simulink model "Ground_Path"  (R2018a)
settings: Solver=ode1  StartTime=0.0  StopTime=constants.t_end  FixedStep=constants.dt  RelTol=1e-3  EnableMultiTasking=on
settings Model: ExtModeTrigDuration=5000  Creator=bruders  LastModifiedBy=Joseph
settings SolverCC: PositivePriorityOrder=on
settings DataIOCC: LimitDataPoints=on  SaveFormat=Array
settings OptimizationCC: LifeSpan=inf
settings DebuggingCC: SolverPrmCheckMsg=warning  AllowSymbolicDim=off  SFUnexpectedBacktrackingDiag=warning  SFNoUnconditionalDefaultTransitionDiag=warning  SFExecutionAtInitializationDiag=none
settings HardwareCC: ProdBitPerPointer=32  ProdBitPerSizeT=32  ProdBitPerPtrDiffT=32  ProdLargestAtomicFloat=None  ProdIntDivRoundTo=Undefined  ProdEndianess=Unspecified  ProdWordSize=32  ProdHWDeviceType=32-bit Generic
settings ModelReferenceCC: PropagateSignalLabelsOutOfModel=off
settings RTWCC: Description=QUARC Win64 Target  SystemTargetFile=quarc_win64.tlc  TemplateMakefile=quarc_default_tmf
settings CodeAppCC: StateflowObjectComments=on
settings STFCustomTargetCC: TargetPreCompLibLocation=C:\PROGRA~3\QUARC\lib\2016b\win64\release  ConcurrentExecutionCompliant=on  GeneratePreprocessorConditionals=Disable all  SystemTargetFile=quarc_win64.tlc
settings GRTTargetCC: TargetPreCompLibLocation=C:\PROGRA~3\QUARC\lib\2016b\win64\release  TargetLangStandard=C89/C90 (ANSI)  ParMdlRefBuildCompliant=off  CompOptLevelCompliant=off  GeneratePreprocessorConditionals=Disable all  CombineOutputUpdateFcns=off  MatFileLogging=off  CPPClassGenCompliant=off  GRTInterface=on  UseToolchainInfoCompliant=off  ExtMode=on  ExtModeMexFile=quarc_comm
settings ConfigComp: CovMetricSettings=dw  CovHtmlReporting=on  CovSaveCumulativeToWorkspaceVar=on  CovSaveSingleToWorkspaceVar=on  CovExternalEMLEnable=off  CovSFcnEnable=off

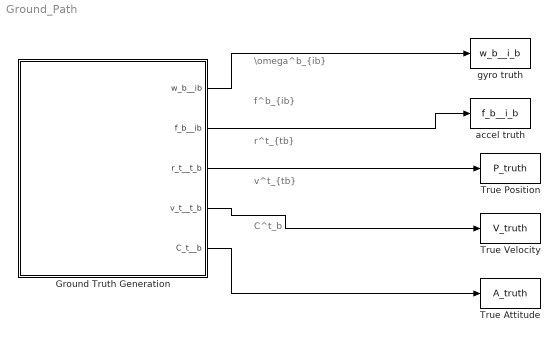
== system Ground_Path ==
  note: f^b_{ib}
  note: \omega^b_{ib}
  note: C^t_b
  note: v^t_{tb}
  note: r^t_{tb}
  Ground Truth Generation : Subsystem
      mask Display: image('Gnd_truth.jpg');
  True Attitude : ToWorkspace  VariableName=A_truth  SampleTime=-1
  True Position : ToWorkspace  VariableName=P_truth  SampleTime=-1
  True Velocity : ToWorkspace  VariableName=V_truth  SampleTime=-1
  accel truth : ToWorkspace  VariableName=f_b__i_b  SampleTime=-1
  gyro truth : ToWorkspace  VariableName=w_b__i_b  SampleTime=-1
  wires:
  Ground Truth Generation/1(w_b__ib) -> gyro truth/1
  Ground Truth Generation/2(f_b__ib) -> accel truth/1
  Ground Truth Generation/3(r_t__t_b) -> True Position/1
  Ground Truth Generation/4(v_t__t_b) -> True Velocity/1
  Ground Truth Generation/5(C_t__b) -> True Attitude/1

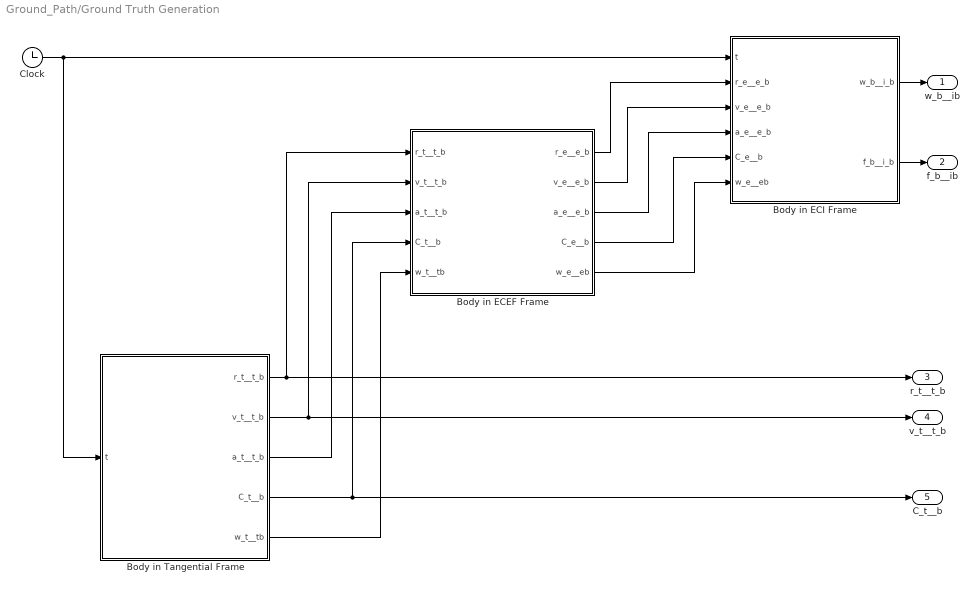
== system Ground_Path/Ground Truth Generation ==
  Body in ECEF Frame : MATLAB Function  TreatAsAtomicUnit=on
  Body in ECI Frame : MATLAB Function  TreatAsAtomicUnit=on
  Body in Tangential Frame : MATLAB Function  TreatAsAtomicUnit=on
  Clock : Clock
  w_b__ib : Outport  VectorParamsAs1DForOutWhenUnconnected=off
  f_b__ib : Outport  Port=2  VectorParamsAs1DForOutWhenUnconnected=off
  r_t__t_b : Outport  Port=3  VectorParamsAs1DForOutWhenUnconnected=off
  v_t__t_b : Outport  Port=4  VectorParamsAs1DForOutWhenUnconnected=off
  C_t__b : Outport  Port=5  VectorParamsAs1DForOutWhenUnconnected=off
  wires:
  Clock/1 -> Body in Tangential Frame/1(t), Body in ECI Frame/1(t)
  Body in Tangential Frame/1(r_t__t_b) -> Body in ECEF Frame/1(r_t__t_b), r_t__t_b/1
  Body in Tangential Frame/2(v_t__t_b) -> Body in ECEF Frame/2(v_t__t_b), v_t__t_b/1
  Body in Tangential Frame/4(C_t__b) -> C_t__b/1, Body in ECEF Frame/4(C_t__b)
  Body in Tangential Frame/3(a_t__t_b) -> Body in ECEF Frame/3(a_t__t_b)
  Body in ECEF Frame/1(r_e__e_b) -> Body in ECI Frame/2(r_e__e_b)
  Body in ECEF Frame/2(v_e__e_b) -> Body in ECI Frame/3(v_e__e_b)
  Body in ECEF Frame/3(a_e__e_b) -> Body in ECI Frame/4(a_e__e_b)
  Body in ECEF Frame/4(C_e__b) -> Body in ECI Frame/5(C_e__b)
  Body in Tangential Frame/5(w_t__tb) -> Body in ECEF Frame/5(w_t__tb)
  Body in ECI Frame/1(w_b__i_b) -> w_b__ib/1
  Body in ECEF Frame/5(w_e__eb) -> Body in ECI Frame/6(w_e__eb)
  Body in ECI Frame/2(f_b__i_b) -> f_b__ib/1

== matlab function Ground_Path/Ground Truth Generation/Body in ECEF Frame ==
  data: r_t__t_b input; v_t__t_b input; a_t__t_b input; C_t__b input; w_t__tb input; r_e__e_b output; constants parameter; v_e__e_b output; a_e__e_b output; C_e__b output; w_e__eb output
function [r_e__e_b, v_e__e_b, a_e__e_b, C_e__b, w_e__eb] = Tan_to_ECEF(r_t__t_b, v_t__t_b, a_t__t_b, C_t__b, w_t__tb, constants)
%#codegen
%
% FUNCTION DESCRIPTION:
%   Propagates quantities from the NAV to BODY coordinate frame
%
% INPUTS:
%   r_t__t_b = Position         of {b} wrt {t} resolved in {t} (m)
%   v_t__t_b = Velocity         of {b} wrt {t} resolved in {t} (m/s)
%   a_t__t_b = Acceleration     of {b} wrt {t} resolved in {t} (m/s^2)
%   C_t__b   = Attitude         of the b-frame wrt the t-frame
%   w_t__tb  = Angular Velocity of {b} wrt {t} resolved in {t} (rad/s)
%   constants= A structure containing various constant parameters
%
% OUTPUTS:
%   r_e__e_b = Position         of {b} wrt {e} resolved in {e} (m)
%   v_e__e_b = Velocity         of {b} wrt {e} resolved in {e} (m/s)
%   a_e__e_b = Acceleration     of {b} wrt {e} resolved in {e} (m/s^2)
%   C_e__b   = Attitude         of the b-frame wrt the e-frame
%   w_e__eb  = Angular Velocity of {b} wrt {e} resolved in {e} (rad/s)
%
% NOTES:
%   - None
%
% REFERENCE:
%   http://mercury.pr.erau.edu/~bruders EE 440 Modern Navigation

% Position of the t-frame wrt the e-frame resolved in {e} (m) - A constant vector
r_e__e_t = constants.r_e__e_t;

% Orientation/Attitude of the Tangential-frame wrt the ECEF-frame
C_e__t = constants.C_e__t ;

% Position of the b-frame wrt the e-frame resolved in {e} (m)
r_e__e_b = r_e__e_t + C_e__t * r_t__t_b;

% Velocity of the b-frame wrt the e-frame resolved in {e} (m/s)
v_e__e_b = C_e__t * v_t__t_b;
       
% Acceleration of the b-frame wrt the e-frame resolved in {e} (m/s^2)
a_e__e_b = C_e__t * a_t__t_b;
        
% Orientation/Attitude of the Body-frame wrt the ECEF-frame
 C_e__b = C_e__t * C_t__b;         

% Angular velocity of the b-frame wrt the e-frame resolved in {e} (rad/s)
w_e__eb = C_e__t * w_t__tb;

== matlab function Ground_Path/Ground Truth Generation/Body in ECI Frame ==
  data: t input; r_e__e_b input; v_e__e_b input; a_e__e_b input; C_e__b input; w_e__eb input; constants parameter; w_b__i_b output; f_b__i_b output
function [w_b__i_b, f_b__i_b] = ECEF_to_ECI(t, r_e__e_b, v_e__e_b, a_e__e_b, C_e__b, w_e__eb, constants)
%#codegen
%
% FUNCTION DESCRIPTION:
%   Propagates quantities from the NAV to BODY coordinate frame
%
% INPUTS:
%   r_e__e_b = Position         of {b} wrt {e} resolved in {e} (m)
%   v_e__e_b = Velocity         of {b} wrt {e} resolved in {e} (m/s)
%   a_e__e_b = Acceleration     of {b} wrt {e} resolved in {e} (m/s^2)
%   C_e__b   = Attitude         of the b-frame wrt the e-frame
%   w_e__eb  = Angular Velocity of {b} wrt {e} resolved in {e} (rad/s)
%   constants= A structure containing various constant parameters
%
% OUTPUTS:
%   w_i__i_b = Angular velocity of {b} wrt {i} resolved in {i} (rad/s)
%   a_i__i_b = Acceleration     of {b} wrt {i} resolved in {i} (m/s^2)
%
% NOTES:
%   - None
%
% REFERENCE:
%   http://mercury.pr.erau.edu/~bruders EE 440 Modern Navigation

w_i__i_e   = constants.w_i__i_e;            % Angular velocity of {e} wrt {i} resolved in {i} (rad/s)
Ohm_i__i_e = constants.Ohm_i__i_e;          % Skew symmetric version of w_i__i_e (rad/s)

% Generate Orientation (i.e., Attitude)
theta_e = constants.w_ie * t + 0;           % Rotational angle theta_e = w_ie t + theta_GMST

C_i__e = [ cos(theta_e), -sin(theta_e), 0   % Orientation of {e} wrt {i}
           sin(theta_e),  cos(theta_e), 0
           0           , 0            , 1];

% Position of the b-frame wrt the i-frame resolved in {i} (m)
r_i__i_b = C_i__e * r_e__e_b;

% Velocity of the b-frame wrt the i-frame resolved in {i} (m/s)
v_i__i_b = C_i__e * (v_e__e_b + Ohm_i__i_e * r_e__e_b);
       
% Acceleration of the b-frame wrt the i-frame resolved in {i} (m/s^2)
a_i__i_b = C_i__e * (a_e__e_b + 2*Ohm_i__i_e * v_e__e_b + Ohm_i__i_e * Ohm_i__i_e * r_e__e_b);
        
% Orientation/Attitude of the Body-frame wrt the ECI-frame
C_i__b = C_i__e * C_e__b;     

% Angular velocity: Ideal Gyro Measurements
w_b__i_b = C_i__b' * (w_i__i_e + C_i__e * w_e__eb);       % Ideal gyro measurements

% Specific Force: Ideal Accel Measurements
[L_b, lambda_b, h_b] = xyz2llh(r_e__e_b, constants);    % Compute the lat, lon, and height of body
g_n__b = [0; 0; gravity(L_b, h_b, constants)];          % Compute the acceleration due to gravity
C_e__n = Lat_Lon_2C_e__n(L_b, lambda_b);                % Compute C_e__n
g_e__b = C_e__n * g_n__b;                               % Compute the gravity of the body in the {e} frame
f_b__i_b = C_i__b' * (a_i__i_b - C_i__e * g_e__b - Ohm_i__i_e * Ohm_i__i_e * r_i__i_b);      % Ideal accel measurements

== matlab function Ground_Path/Ground Truth Generation/Body in Tangential Frame ==
  data: t input; r_t__t_b output; constants parameter; v_t__t_b output; a_t__t_b output; C_t__b output; w_t__tb output
function [r_t__t_b, v_t__t_b, a_t__t_b, C_t__b, w_t__tb] = Body_in_Tan(t, constants)
%#codegen
%
% FUNCTION DESCRIPTION:
%   Propagates quantities from the NAV to BODY coordinate frame
%
% INPUTS:
%   t_sec    = Time (sec)
%   constants= A structure containing various constant parameters
%
% OUTPUTS:
%   r_t__t_b = Position         of {b} wrt {t} resolved in {t} (m)
%   v_t__t_b = Velocity         of {b} wrt {t} resolved in {t} (m/s)
%   a_t__t_b = Acceleration     of {b} wrt {t} resolved in {t} (m/s^2)
%   C_t__b   = Attitude         of the b-frame wrt the t-frame (dimless)
%   w_t__tb  = Angular Velocity of {b} wrt {t} resolved in {t} (rad/s)
% NOTES:
%   - None
%
% REFERENCE:
%   http://mercury.pr.erau.edu/~bruders EE 440 Modern Navigation

persistent cnt C_t__bm

dT = constants.dt;                  % Sample interval (sec)

Tx = constants.t_end;               % Period of the figure eight (sec) 
fx = 1/Tx;                          % Freq of the Fig eight (Hz)
wx = 4*pi*fx;                       % Freq of the Fig eight (rad/s)

Ax = 20;                            % Amplitude of fig eight in x-dir
Ay = 100;                           % Amplitude of fig eight in y-dir
Az = 50;                            % Amplitude of fig eight in z-dir

% Position of the b-frame wrt the t-frame resolved in {t} (m)
r_t__t_b = [ Ax      * sin(wx*t)   % A North-East-Down (NED) frame
            -Ay      * sin((wx/2)*t)
            -Az      * sin((wx/4)*t)];

% Velocity of the b-frame wrt the t-frame resolved in {t} (m)
v_t__t_b = [ Ax*wx   * cos(wx*t)        % A North-East-Down (NED) frame
            -Ay*wx/2 * cos(t*wx/2)
            -Az*wx/4 * cos(t*wx/4)];  
       
% Accel of the org of the b-frame wrt the t-frame described in the t-frame
a_t__t_b = [-Ax*wx^2    * sin(wx*t)     % A North-East-Down (NED) frame
             Ay*wx^2/4  * sin(t*wx/2)
             Az*wx^2/16 * sin(t*wx/4)];       
        
% Orientation of the b-frame wrt the t-frame (a forward-right-down frame)
x_axis = v_t__t_b / norm(v_t__t_b);     % x-axis points "forward"
% See generic form of the RPY matrix
pitch = asin(-x_axis(3));               % pitch angle (rad)
roll  = 0;
yaw   = atan2(x_axis(2), x_axis(1));    % yaw angle (rad)
C_t__b = ypr2dcm(yaw, pitch, roll);

% Add some roll based on the y-axis accel in the body frame
a_temp = C_t__b' * a_t__t_b;
roll = atan2(a_temp(2), 10);            % Relative to ~g
C_t__b = ypr2dcm(yaw, pitch, roll);     % Update DCM        
 
if isempty(cnt) % First time into the function?
    w_t__tb = [0;0;0];  % Initialize at 0
    cnt = 1;            % Any value will do
    C_t__bm = eye(3);
else
    %% THis method of generating w from C has the undesired effect of
    %% causing the low-fidelity mech to be more accurate than the high!!!
    %% Change the way
%     C_t__b_dot = (C_t__b - C_t__bm)/dT; % C_dot
%     Ohm_t__tb = C_t__b_dot * C_t__b';   % OHM = C_dot C'
%     w_t__tb = ss2vec(Ohm_t__tb);        % OHM -> w
    Delta_C = C_t__b * C_t__bm';    % C_t__b(k) = exp(OHMC_t__tb*dT) C_t__b(k-1)
    w_t__tb = dcm2k(Delta_C) / dT;  % C_t__b(k) = C_t__b(k-1) exp(OHMC_b__tb*dT)
end
C_t__bm = C_t__b;   % Store the current DCM for use in the next iteration
